simulink model "Correlation_Ex2"  (R2024a)
settings: Solver=VariableStepAuto  StartTime=0.0  StopTime=1024/100e6  RelTol=1e-3
undefined symbols (not defined in the file): S, vsva2197, xcvc1902
libraries: dspsrcs4 x2, aieDSP x1, dspstat3 x1, vmcUtilities x1
settings Model: Creator=sdegala  LastModifiedBy=robg

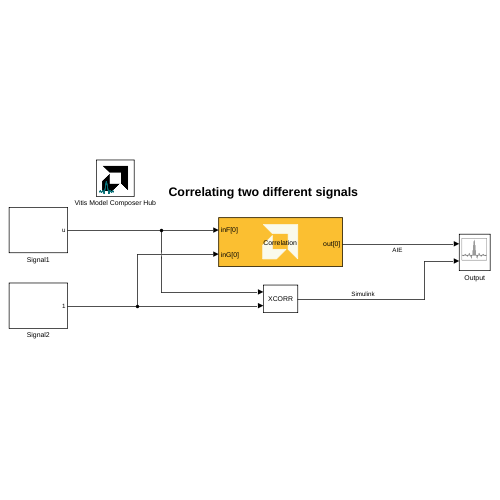
[thumbnail: Simulink's stored preview of the top-level diagram]
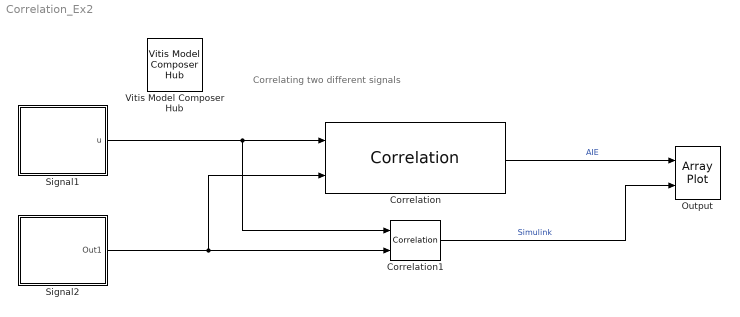
== system Correlation_Ex2 ==
  note: Correlating two different signals
  Correlation : aieDSP/Correlation  AIE_VARIANT=1  api=0  data_type_f=float  data_type_g=float  data_type_out=float  function_type=0  compute_mode=Full  f_sample_size=32  g_sample_size=32  USE_RTP_VECTOR_LENGTHS=off  num_frames=1  shift_output=0  rnd_mode=Floor  sat_mode=None  no_of_kernels=1  casc_length=1  blockJsonConstraints=[]  blockJsonConstraintsInternal=[]  spec=vmc_corr.json  SerializedMaskParamNames=[]  SerializedMaskParamValues=[]  SerializedMaskParamVisibilities=[]  block_type=Correlation  SerializedMaskParamDataypes=uint|uint|typename|typename|typename|uint|uint|uint|uint|uint|uint|uint|uint|uint|uint|uint  SerializedMaskParamEnumStrArr=0|0|0|0|0|0|Full,Same,Valid|0|0|0|0|0|Floor,Ceiling,Round to positive infinity,Round to negative infinity,Round symmetrical to infinity,Round symmetrical to zero,Round convergent to even,Round convergent to odd|None,Saturate,Symmetric|0|0  SerializedMaskParamEnumValArr=0|0|0|0|0|0|0,1,2|0|0|0|0|0|0,1,2,3,4,5,6,7|0,1,3|0|0  SerializedMaskParamVectorArr=0|0|0|0|0|0|0|0|0|0|0|0|0|0|0|0  SerializedMaskParamKeys=AIE_VARIANT|TP_API|TT_DATA_F|TT_DATA_G|TT_DATA_OUT|TP_FUNCT_TYPE|TP_COMPUTE_MODE|TP_F_LEN|TP_G_LEN|TP_USE_RTP_VECTOR_LENGTHS|TP_NUM_FRAMES|TP_SHIFT|TP_RND|TP_SAT|TP_PHASES|TP_CASC_LEN
  Correlation1 : dspstat3/Correlation  domain=Time  roundingMode=Floor  overflowMode=off  outputDataTypeStr=Inherit: Same as accumulator  outputMin=[]  outputMax=[]  outputLastDataTypeStr=Inherit: Same as accumulator
  Output : ArrayPlot  NumInputPorts=2  WindowPosition=[1021.000000,450.000000,800.000000,516.000000,]  Visible=on  ScopeFrameLocation=window  YLimits=[-12.6852 1.8596]  ShowLegend=on
  Signal1 : Subsystem
  Signal2 : Subsystem
  Vitis Model Composer Hub : vmcUtilities/Vitis Model Composer Hub  Tag=genX  CodeGeneration=off  StartColumn=1  NumberOfColumns=1  TargetDirectory=./code  exportDesign=off  analyzeDesign=off  validateDesignOnHw=off  ExportType=AI Engines  IpVendor=xilinx.com  IpLibrary=hls  IpVersion=1.0  IpHWLanguage=Verilog  AieCompilerOptions={}  AieSimulatorOptions={}  CreateTestbench=off  TestbenchStackSize=10  RunRtlSim=off  RunCSim=off  RunAieSim=off  AieSimTimeout=50000  RunAieSimProfiling=off  LaunchVitisAnalyzer=off  PlotOutput=off  RunX86Sim=off  X86SimTimeout=10  GenHwImage=off  GenLibadfXo=off  GenHwValidationCode=off  PlatformType=Not Specified  HwSystemType=Baremetal  HwValidationTarget=hw  ProjDevice=xcvc1902-vsva2197-1LP-e-S  ProjDevicePart=xcvc1902-vsva2197-1LP-e-S  AIEType=AIE  SamplePeriod=-1  ClockFrequency=200  DataPathParallelism=1  xilinxfamily=versalaicore  part=xcvc1902  speed=-1LP-e-S  package=vsva2197  directory=./netlist  testbench=off  incr_netlist=off  synthesis_tool=Vivado  clock_wrapper=Clock Enables  dbl_ovrd=According to Block Masks  dcm_input_clock_period=10  sysclk_period=10  simulink_period=1  eval_field=0  LogFileName=''  NThreads=4
  wires:
  Signal2/1(Out1) -> Correlation1/2, Correlation/2
  Correlation1/1 -> Output/2  "Simulink"
  Correlation/1 -> Output/1  "AIE"
  Signal1/1(u) -> Correlation1/1, Correlation/1

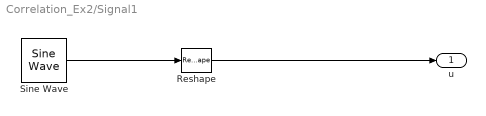
== system Correlation_Ex2/Signal1 ==
  Reshape : Reshape
  Sine Wave : dspsrcs4/Sine Wave  Amplitude=1  Frequency=1e6  Phase=0  SampleMode=Discrete  OutComplex=Real  CompMethod=Trigonometric fcn  TableSize=Speed  SampleTime=1/100e6  SamplesPerFrame=32  ResetState=Restart at time zero  OutputFrames=off  dataType=single  wordLen=16  udDataType=sfix(16)  fracBitsMode=Best precision  numFracBits=15  OutDataTypeStr=single  LastOutDataTypeStr=single
  u : Outport
  wires:
  Sine Wave/1 -> Reshape/1
  Reshape/1 -> u/1

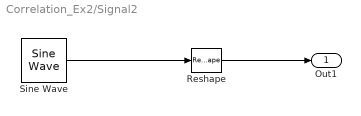
== system Correlation_Ex2/Signal2 ==
  Reshape : Reshape
  Sine Wave : dspsrcs4/Sine Wave  Amplitude=5  Frequency=50e3  Phase=0  SampleMode=Discrete  OutComplex=Real  CompMethod=Trigonometric fcn  TableSize=Speed  SampleTime=1/100e6  SamplesPerFrame=32  ResetState=Restart at time zero  OutputFrames=off  dataType=single  wordLen=16  udDataType=sfix(16)  fracBitsMode=Best precision  numFracBits=15  OutDataTypeStr=single  LastOutDataTypeStr=single
  Out1 : Outport
  wires:
  Sine Wave/1 -> Reshape/1
  Reshape/1 -> Out1/1
